simulink model "modern2"  (R2024b)
settings: Solver=VariableStepAuto  StartTime=0.0  StopTime=50  RelTol=1e-3
undefined symbols (not defined in the file): b1, b2, K1, K2, M1, M2
settings Model: LastModifiedBy=ARVIND TRIVEDI

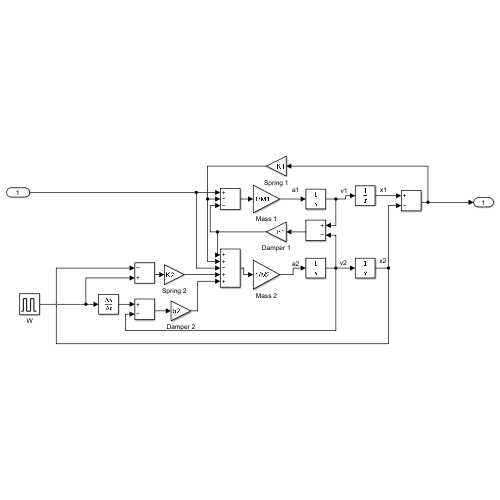
[thumbnail: Simulink's stored preview of the top-level diagram]
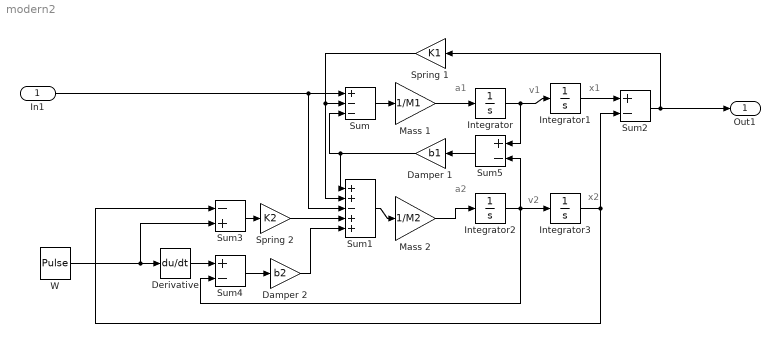
== system modern2 ==
  note: a1
  note: v1
  note: v2
  note: x2
  note: a2
  note: x1
  In1 : Inport
  Damper 1 : Gain  Gain=b1  SaturateOnIntegerOverflow=on  OutDataTypeStr=Inherit: Same as input  ParamDataTypeStr=Inherit: Same as input
  Damper 2 : Gain  Gain=b2  SaturateOnIntegerOverflow=on  OutDataTypeStr=Inherit: Same as input  ParamDataTypeStr=Inherit: Same as input
  Derivative : Derivative
  Integrator{,1..3} (4 alike) : Integrator
  Mass 1 : Gain  Gain=1/M1  SaturateOnIntegerOverflow=on  OutDataTypeStr=Inherit: Same as input  ParamDataTypeStr=Inherit: Same as input
  Mass 2 : Gain  Gain=1/M2  SaturateOnIntegerOverflow=on  OutDataTypeStr=Inherit: Same as input  ParamDataTypeStr=Inherit: Same as input
  Spring 1 : Gain  Gain=K1  SaturateOnIntegerOverflow=on  OutDataTypeStr=Inherit: Same as input  ParamDataTypeStr=Inherit: Same as input
  Spring 2 : Gain  Gain=K2  SaturateOnIntegerOverflow=on  OutDataTypeStr=Inherit: Same as input  ParamDataTypeStr=Inherit: Same as input
  Sum : Sum  Inputs=+--  InputSameDT=on  SaturateOnIntegerOverflow=on  OutDataTypeStr=Inherit: Same as first input
  Sum1 : Sum  Inputs=++-++  InputSameDT=on  SaturateOnIntegerOverflow=on  OutDataTypeStr=Inherit: Same as first input
  Sum2 : Sum  Inputs=+-  InputSameDT=on  SaturateOnIntegerOverflow=on  OutDataTypeStr=Inherit: Same as first input
  Sum3 : Sum  Inputs=-+  InputSameDT=on  SaturateOnIntegerOverflow=on  OutDataTypeStr=Inherit: Same as first input
  Sum4 : Sum  Inputs=+-  InputSameDT=on  SaturateOnIntegerOverflow=on  OutDataTypeStr=Inherit: Same as first input
  Sum5 : Sum  Inputs=+-  InputSameDT=on  SaturateOnIntegerOverflow=on  OutDataTypeStr=Inherit: Same as first input
  W : DiscretePulseGenerator  PulseType=Time based  Period=100  PulseWidth=0.1
  Out1 : Outport
  wires:
  Integrator2/1 -> Integrator3/1, Sum4/2, Sum5/2
  Spring 1/1 -> Sum/2, Sum1/2
  Sum1/1 -> Mass 2/1
  Damper 2/1 -> Sum1/5
  Mass 2/1 -> Integrator2/1
  Sum5/1 -> Damper 1/1
  Sum4/1 -> Damper 2/1
  Spring 2/1 -> Sum1/4
  W/1 -> Sum3/2, Derivative/1
  Mass 1/1 -> Integrator/1
  Integrator3/1 -> Sum2/2, Sum3/1
  In1/1 -> Sum1/3, Sum/1
  Sum2/1 -> Out1/1, Spring 1/1
  Sum3/1 -> Spring 2/1
  Integrator1/1 -> Sum2/1
  Integrator/1 -> Integrator1/1, Sum5/1
  Damper 1/1 -> Sum1/1, Sum/3
  Sum/1 -> Mass 1/1
  Derivative/1 -> Sum4/1
